simulink model "c00009M_harness"  (R2018a)
settings: Solver=FixedStepAuto  StartTime=0.0  StopTime=300  FixedStep=0.1  RelTol=1e-3
undefined symbols (not defined in the file): A1, hmax, PriorityTank, R1, R2, sigbuilder_block
(part 8 of 29)

== system c00009M_harness/M090/Tank2 ==
  CT2 : Inport
  MR2 : Inport  Port=2
  T2 : Inport  Port=3
  EB2 : Inport  Port=4
  LL1 : Inport  Port=5
  Control : Subsystem
  Logical Operator : Logic  AllPortsSameDT=off  OutDataTypeStr=boolean
  MasterTankControl : Subsystem
  Memory : Memory
  Memory1 : Memory
  TankModel : Subsystem
  LL2 : Outport
  wires:
  TankModel/1(LiquidLevel) -> Memory/1, LL2/1
  Control/1(LiquidIn) -> Logical Operator/1
  Control/2(LiquidOut) -> TankModel/2(LiquidOut)
  Memory/1 -> Control/5(LiquidLevel), MasterTankControl/2(LiquidTank2)
  MR2/1 -> Control/3(ManualReference)
  CT2/1 -> Control/2(StartMaintenance), Control/1(ControlType)
  Memory1/1 -> MasterTankControl/1(LiquidTank1)
  EB2/1 -> Control/4(EmergencyButton)
  MasterTankControl/1(AllowTheTankFilling) -> Logical Operator/2
  Logical Operator/1 -> TankModel/1(LiquidIn)
  LL1/1 -> Memory1/1

== system c00009M_harness/M091/Tank1 ==
  CT1 : Inport
  MR1 : Inport  Port=2
  T1 : Inport  Port=3
  EB1 : Inport  Port=4
  LL2 : Inport  Port=5
  Control : Subsystem
  Logical Operator : Logic  AllPortsSameDT=off  OutDataTypeStr=boolean
  MasterTankControl : Subsystem
  Memory : Memory
  Memory1 : Memory
  TankModel : Subsystem
  LL1 : Outport
  wires:
  TankModel/1(LiquidLevel) -> Memory/1, LL1/1
  Control/1(LiquidIn) -> Logical Operator/1
  Control/2(LiquidOut) -> TankModel/2(LiquidOut)
  Memory/1 -> Control/4(LiquidLevel), MasterTankControl/1(LiquidTank1)
  MR1/1 -> Control/2(ManualReference)
  CT1/1 -> Control/1(ControlType)
  Memory1/1 -> MasterTankControl/2(LiquidTank2)
  EB1/1 -> Control/3(EmergencyButton)
  MasterTankControl/1(AllowTheTankFilling) -> Logical Operator/2
  Logical Operator/1 -> TankModel/1(LiquidIn)
  LL2/1 -> Memory1/1

== system c00009M_harness/M091/Tank2 ==
  CT2 : Inport
  MR2 : Inport  Port=2
  T2 : Inport  Port=3
  EB2 : Inport  Port=4
  LL1 : Inport  Port=5
  Control : Subsystem
  Logical Operator : Logic  AllPortsSameDT=off  OutDataTypeStr=boolean
  MasterTankControl : Subsystem
  Memory : Memory
  Memory1 : Memory
  TankModel : Subsystem
  LL2 : Outport
  wires:
  TankModel/1(LiquidLevel) -> Memory/1, LL2/1
  Control/1(LiquidIn) -> Logical Operator/1
  Control/2(LiquidOut) -> TankModel/2(LiquidOut)
  Memory/1 -> Control/5(LiquidLevel), MasterTankControl/2(LiquidTank2)
  MR2/1 -> Control/3(ManualReference)
  CT2/1 -> Control/2(StartMaintenance), Control/1(ControlType)
  Memory1/1 -> MasterTankControl/1(LiquidTank1)
  EB2/1 -> Control/4(EmergencyButton)
  MasterTankControl/1(AllowTheTankFilling) -> Logical Operator/2
  Logical Operator/1 -> TankModel/1(LiquidIn)
  LL1/1 -> Memory1/1

== system c00009M_harness/M092/Tank1 ==
  CT1 : Inport
  MR1 : Inport  Port=2
  T1 : Inport  Port=3
  EB1 : Inport  Port=4
  LL2 : Inport  Port=5
  Control : Subsystem
  Logical Operator : Logic  AllPortsSameDT=off  OutDataTypeStr=boolean
  MasterTankControl : Subsystem
  Memory : Memory
  Memory1 : Memory
  TankModel : Subsystem
  LL1 : Outport
  wires:
  TankModel/1(LiquidLevel) -> Memory/1, LL1/1
  Control/1(LiquidIn) -> Logical Operator/1
  Control/2(LiquidOut) -> TankModel/2(LiquidOut)
  Memory/1 -> Control/4(LiquidLevel), MasterTankControl/1(LiquidTank1)
  MR1/1 -> Control/2(ManualReference)
  CT1/1 -> Control/1(ControlType)
  Memory1/1 -> MasterTankControl/2(LiquidTank2)
  EB1/1 -> Control/3(EmergencyButton)
  MasterTankControl/1(AllowTheTankFilling) -> Logical Operator/2
  Logical Operator/1 -> TankModel/1(LiquidIn)
  LL2/1 -> Memory1/1

== system c00009M_harness/M092/Tank2 ==
  CT2 : Inport
  MR2 : Inport  Port=2
  T2 : Inport  Port=3
  EB2 : Inport  Port=4
  LL1 : Inport  Port=5
  Control : Subsystem
  Logical Operator : Logic  AllPortsSameDT=off  OutDataTypeStr=boolean
  MasterTankControl : Subsystem
  Memory : Memory
  Memory1 : Memory
  TankModel : Subsystem
  LL2 : Outport
  wires:
  TankModel/1(LiquidLevel) -> Memory/1, LL2/1
  Control/1(LiquidIn) -> Logical Operator/1
  Control/2(LiquidOut) -> TankModel/2(LiquidOut)
  Memory/1 -> Control/5(LiquidLevel), MasterTankControl/2(LiquidTank2)
  MR2/1 -> Control/3(ManualReference)
  CT2/1 -> Control/2(StartMaintenance), Control/1(ControlType)
  Memory1/1 -> MasterTankControl/1(LiquidTank1)
  EB2/1 -> Control/4(EmergencyButton)
  MasterTankControl/1(AllowTheTankFilling) -> Logical Operator/2
  Logical Operator/1 -> TankModel/1(LiquidIn)
  LL1/1 -> Memory1/1

== system c00009M_harness/M093/Tank1 ==
  CT1 : Inport
  MR1 : Inport  Port=2
  T1 : Inport  Port=3
  EB1 : Inport  Port=4
  LL2 : Inport  Port=5
  Control : Subsystem
  Logical Operator : Logic  AllPortsSameDT=off  OutDataTypeStr=boolean
  MasterTankControl : Subsystem
  Memory : Memory
  Memory1 : Memory
  TankModel : Subsystem
  LL1 : Outport
  wires:
  TankModel/1(LiquidLevel) -> Memory/1, LL1/1
  Control/1(LiquidIn) -> Logical Operator/1
  Control/2(LiquidOut) -> TankModel/2(LiquidOut)
  Memory/1 -> Control/4(LiquidLevel), MasterTankControl/1(LiquidTank1)
  MR1/1 -> Control/2(ManualReference)
  CT1/1 -> Control/1(ControlType)
  Memory1/1 -> MasterTankControl/2(LiquidTank2)
  EB1/1 -> Control/3(EmergencyButton)
  MasterTankControl/1(AllowTheTankFilling) -> Logical Operator/2
  Logical Operator/1 -> TankModel/1(LiquidIn)
  LL2/1 -> Memory1/1

== system c00009M_harness/M093/Tank2 ==
  CT2 : Inport
  MR2 : Inport  Port=2
  T2 : Inport  Port=3
  EB2 : Inport  Port=4
  LL1 : Inport  Port=5
  Control : Subsystem
  Logical Operator : Logic  AllPortsSameDT=off  OutDataTypeStr=boolean
  MasterTankControl : Subsystem
  Memory : Memory
  Memory1 : Memory
  TankModel : Subsystem
  LL2 : Outport
  wires:
  TankModel/1(LiquidLevel) -> Memory/1, LL2/1
  Control/1(LiquidIn) -> Logical Operator/1
  Control/2(LiquidOut) -> TankModel/2(LiquidOut)
  Memory/1 -> Control/5(LiquidLevel), MasterTankControl/2(LiquidTank2)
  MR2/1 -> Control/3(ManualReference)
  CT2/1 -> Control/2(StartMaintenance), Control/1(ControlType)
  Memory1/1 -> MasterTankControl/1(LiquidTank1)
  EB2/1 -> Control/4(EmergencyButton)
  MasterTankControl/1(AllowTheTankFilling) -> Logical Operator/2
  Logical Operator/1 -> TankModel/1(LiquidIn)
  LL1/1 -> Memory1/1

== system c00009M_harness/M094/Tank1 ==
  CT1 : Inport
  MR1 : Inport  Port=2
  T1 : Inport  Port=3
  EB1 : Inport  Port=4
  LL2 : Inport  Port=5
  Control : Subsystem
  Logical Operator : Logic  AllPortsSameDT=off  OutDataTypeStr=boolean
  MasterTankControl : Subsystem
  Memory : Memory
  Memory1 : Memory
  TankModel : Subsystem
  LL1 : Outport
  wires:
  TankModel/1(LiquidLevel) -> Memory/1, LL1/1
  Control/1(LiquidIn) -> Logical Operator/1
  Control/2(LiquidOut) -> TankModel/2(LiquidOut)
  Memory/1 -> Control/4(LiquidLevel), MasterTankControl/1(LiquidTank1)
  MR1/1 -> Control/2(ManualReference)
  CT1/1 -> Control/1(ControlType)
  Memory1/1 -> MasterTankControl/2(LiquidTank2)
  EB1/1 -> Control/3(EmergencyButton)
  MasterTankControl/1(AllowTheTankFilling) -> Logical Operator/2
  Logical Operator/1 -> TankModel/1(LiquidIn)
  LL2/1 -> Memory1/1

== system c00009M_harness/M094/Tank2 ==
  CT2 : Inport
  MR2 : Inport  Port=2
  T2 : Inport  Port=3
  EB2 : Inport  Port=4
  LL1 : Inport  Port=5
  Control : Subsystem
  Logical Operator : Logic  AllPortsSameDT=off  OutDataTypeStr=boolean
  MasterTankControl : Subsystem
  Memory : Memory
  Memory1 : Memory
  TankModel : Subsystem
  LL2 : Outport
  wires:
  TankModel/1(LiquidLevel) -> Memory/1, LL2/1
  Control/1(LiquidIn) -> Logical Operator/1
  Control/2(LiquidOut) -> TankModel/2(LiquidOut)
  Memory/1 -> Control/5(LiquidLevel), MasterTankControl/2(LiquidTank2)
  MR2/1 -> Control/3(ManualReference)
  CT2/1 -> Control/2(StartMaintenance), Control/1(ControlType)
  Memory1/1 -> MasterTankControl/1(LiquidTank1)
  EB2/1 -> Control/4(EmergencyButton)
  MasterTankControl/1(AllowTheTankFilling) -> Logical Operator/2
  Logical Operator/1 -> TankModel/1(LiquidIn)
  LL1/1 -> Memory1/1

== system c00009M_harness/M095/Tank1 ==
  CT1 : Inport
  MR1 : Inport  Port=2
  T1 : Inport  Port=3
  EB1 : Inport  Port=4
  LL2 : Inport  Port=5
  Control : Subsystem
  Logical Operator : Logic  AllPortsSameDT=off  OutDataTypeStr=boolean
  MasterTankControl : Subsystem
  Memory : Memory
  Memory1 : Memory
  TankModel : Subsystem
  LL1 : Outport
  wires:
  TankModel/1(LiquidLevel) -> Memory/1, LL1/1
  Control/1(LiquidIn) -> Logical Operator/1
  Control/2(LiquidOut) -> TankModel/2(LiquidOut)
  Memory/1 -> Control/4(LiquidLevel), MasterTankControl/1(LiquidTank1)
  MR1/1 -> Control/2(ManualReference)
  CT1/1 -> Control/1(ControlType)
  Memory1/1 -> MasterTankControl/2(LiquidTank2)
  EB1/1 -> Control/3(EmergencyButton)
  MasterTankControl/1(AllowTheTankFilling) -> Logical Operator/2
  Logical Operator/1 -> TankModel/1(LiquidIn)
  LL2/1 -> Memory1/1

== system c00009M_harness/M095/Tank2 ==
  CT2 : Inport
  MR2 : Inport  Port=2
  T2 : Inport  Port=3
  EB2 : Inport  Port=4
  LL1 : Inport  Port=5
  Control : Subsystem
  Logical Operator : Logic  AllPortsSameDT=off  OutDataTypeStr=boolean
  MasterTankControl : Subsystem
  Memory : Memory
  Memory1 : Memory
  TankModel : Subsystem
  LL2 : Outport
  wires:
  TankModel/1(LiquidLevel) -> Memory/1, LL2/1
  Control/1(LiquidIn) -> Logical Operator/1
  Control/2(LiquidOut) -> TankModel/2(LiquidOut)
  Memory/1 -> Control/5(LiquidLevel), MasterTankControl/2(LiquidTank2)
  MR2/1 -> Control/3(ManualReference)
  CT2/1 -> Control/2(StartMaintenance), Control/1(ControlType)
  Memory1/1 -> MasterTankControl/1(LiquidTank1)
  EB2/1 -> Control/4(EmergencyButton)
  MasterTankControl/1(AllowTheTankFilling) -> Logical Operator/2
  Logical Operator/1 -> TankModel/1(LiquidIn)
  LL1/1 -> Memory1/1

== system c00009M_harness/M096/Tank1 ==
  CT1 : Inport
  MR1 : Inport  Port=2
  T1 : Inport  Port=3
  EB1 : Inport  Port=4
  LL2 : Inport  Port=5
  Control : Subsystem
  Logical Operator : Logic  AllPortsSameDT=off  OutDataTypeStr=boolean
  MasterTankControl : Subsystem
  Memory : Memory
  Memory1 : Memory
  TankModel : Subsystem
  LL1 : Outport
  wires:
  TankModel/1(LiquidLevel) -> Memory/1, LL1/1
  Control/1(LiquidIn) -> Logical Operator/1
  Control/2(LiquidOut) -> TankModel/2(LiquidOut)
  Memory/1 -> Control/4(LiquidLevel), MasterTankControl/1(LiquidTank1)
  MR1/1 -> Control/2(ManualReference)
  CT1/1 -> Control/1(ControlType)
  Memory1/1 -> MasterTankControl/2(LiquidTank2)
  EB1/1 -> Control/3(EmergencyButton)
  MasterTankControl/1(AllowTheTankFilling) -> Logical Operator/2
  Logical Operator/1 -> TankModel/1(LiquidIn)
  LL2/1 -> Memory1/1

== system c00009M_harness/M096/Tank2 ==
  CT2 : Inport
  MR2 : Inport  Port=2
  T2 : Inport  Port=3
  EB2 : Inport  Port=4
  LL1 : Inport  Port=5
  Control : Subsystem
  Logical Operator : Logic  AllPortsSameDT=off  OutDataTypeStr=boolean
  MasterTankControl : Subsystem
  Memory : Memory
  Memory1 : Memory
  TankModel : Subsystem
  LL2 : Outport
  wires:
  TankModel/1(LiquidLevel) -> Memory/1, LL2/1
  Control/1(LiquidIn) -> Logical Operator/1
  Control/2(LiquidOut) -> TankModel/2(LiquidOut)
  Memory/1 -> Control/5(LiquidLevel), MasterTankControl/2(LiquidTank2)
  MR2/1 -> Control/3(ManualReference)
  CT2/1 -> Control/2(StartMaintenance), Control/1(ControlType)
  Memory1/1 -> MasterTankControl/1(LiquidTank1)
  EB2/1 -> Control/4(EmergencyButton)
  MasterTankControl/1(AllowTheTankFilling) -> Logical Operator/2
  Logical Operator/1 -> TankModel/1(LiquidIn)
  LL1/1 -> Memory1/1

== system c00009M_harness/M097/Tank1 ==
  CT1 : Inport
  MR1 : Inport  Port=2
  T1 : Inport  Port=3
  EB1 : Inport  Port=4
  LL2 : Inport  Port=5
  Control : Subsystem
  Logical Operator : Logic  AllPortsSameDT=off  OutDataTypeStr=boolean
  MasterTankControl : Subsystem
  Memory : Memory
  Memory1 : Memory
  TankModel : Subsystem
  LL1 : Outport
  wires:
  TankModel/1(LiquidLevel) -> Memory/1, LL1/1
  Control/1(LiquidIn) -> Logical Operator/1
  Control/2(LiquidOut) -> TankModel/2(LiquidOut)
  Memory/1 -> Control/4(LiquidLevel), MasterTankControl/1(LiquidTank1)
  MR1/1 -> Control/2(ManualReference)
  CT1/1 -> Control/1(ControlType)
  Memory1/1 -> MasterTankControl/2(LiquidTank2)
  EB1/1 -> Control/3(EmergencyButton)
  MasterTankControl/1(AllowTheTankFilling) -> Logical Operator/2
  Logical Operator/1 -> TankModel/1(LiquidIn)
  LL2/1 -> Memory1/1

== system c00009M_harness/M097/Tank2 ==
  CT2 : Inport
  MR2 : Inport  Port=2
  T2 : Inport  Port=3
  EB2 : Inport  Port=4
  LL1 : Inport  Port=5
  Control : Subsystem
  Logical Operator : Logic  AllPortsSameDT=off  OutDataTypeStr=boolean
  MasterTankControl : Subsystem
  Memory : Memory
  Memory1 : Memory
  TankModel : Subsystem
  LL2 : Outport
  wires:
  TankModel/1(LiquidLevel) -> Memory/1, LL2/1
  Control/1(LiquidIn) -> Logical Operator/1
  Control/2(LiquidOut) -> TankModel/2(LiquidOut)
  Memory/1 -> Control/5(LiquidLevel), MasterTankControl/2(LiquidTank2)
  MR2/1 -> Control/3(ManualReference)
  CT2/1 -> Control/2(StartMaintenance), Control/1(ControlType)
  Memory1/1 -> MasterTankControl/1(LiquidTank1)
  EB2/1 -> Control/4(EmergencyButton)
  MasterTankControl/1(AllowTheTankFilling) -> Logical Operator/2
  Logical Operator/1 -> TankModel/1(LiquidIn)
  LL1/1 -> Memory1/1

== system c00009M_harness/M098/Tank1 ==
  CT1 : Inport
  MR1 : Inport  Port=2
  T1 : Inport  Port=3
  EB1 : Inport  Port=4
  LL2 : Inport  Port=5
  Control : Subsystem
  Logical Operator : Logic  AllPortsSameDT=off  OutDataTypeStr=boolean
  MasterTankControl : Subsystem
  Memory : Memory
  Memory1 : Memory
  TankModel : Subsystem
  LL1 : Outport
  wires:
  TankModel/1(LiquidLevel) -> Memory/1, LL1/1
  Control/1(LiquidIn) -> Logical Operator/1
  Control/2(LiquidOut) -> TankModel/2(LiquidOut)
  Memory/1 -> Control/4(LiquidLevel), MasterTankControl/1(LiquidTank1)
  MR1/1 -> Control/2(ManualReference)
  CT1/1 -> Control/1(ControlType)
  Memory1/1 -> MasterTankControl/2(LiquidTank2)
  EB1/1 -> Control/3(EmergencyButton)
  MasterTankControl/1(AllowTheTankFilling) -> Logical Operator/2
  Logical Operator/1 -> TankModel/1(LiquidIn)
  LL2/1 -> Memory1/1

== system c00009M_harness/M098/Tank2 ==
  CT2 : Inport
  MR2 : Inport  Port=2
  T2 : Inport  Port=3
  EB2 : Inport  Port=4
  LL1 : Inport  Port=5
  Control : Subsystem
  Logical Operator : Logic  AllPortsSameDT=off  OutDataTypeStr=boolean
  MasterTankControl : Subsystem
  Memory : Memory
  Memory1 : Memory
  TankModel : Subsystem
  LL2 : Outport
  wires:
  TankModel/1(LiquidLevel) -> Memory/1, LL2/1
  Control/1(LiquidIn) -> Logical Operator/1
  Control/2(LiquidOut) -> TankModel/2(LiquidOut)
  Memory/1 -> Control/5(LiquidLevel), MasterTankControl/2(LiquidTank2)
  MR2/1 -> Control/3(ManualReference)
  CT2/1 -> Control/2(StartMaintenance), Control/1(ControlType)
  Memory1/1 -> MasterTankControl/1(LiquidTank1)
  EB2/1 -> Control/4(EmergencyButton)
  MasterTankControl/1(AllowTheTankFilling) -> Logical Operator/2
  Logical Operator/1 -> TankModel/1(LiquidIn)
  LL1/1 -> Memory1/1

== system c00009M_harness/M099/Tank1 ==
  CT1 : Inport
  MR1 : Inport  Port=2
  T1 : Inport  Port=3
  EB1 : Inport  Port=4
  LL2 : Inport  Port=5
  Control : Subsystem
  Logical Operator : Logic  AllPortsSameDT=off  OutDataTypeStr=boolean
  MasterTankControl : Subsystem
  Memory : Memory
  Memory1 : Memory
  TankModel : Subsystem
  LL1 : Outport
  wires:
  TankModel/1(LiquidLevel) -> Memory/1, LL1/1
  Control/1(LiquidIn) -> Logical Operator/1
  Control/2(LiquidOut) -> TankModel/2(LiquidOut)
  Memory/1 -> Control/4(LiquidLevel), MasterTankControl/1(LiquidTank1)
  MR1/1 -> Control/2(ManualReference)
  CT1/1 -> Control/1(ControlType)
  Memory1/1 -> MasterTankControl/2(LiquidTank2)
  EB1/1 -> Control/3(EmergencyButton)
  MasterTankControl/1(AllowTheTankFilling) -> Logical Operator/2
  Logical Operator/1 -> TankModel/1(LiquidIn)
  LL2/1 -> Memory1/1

== system c00009M_harness/M099/Tank2 ==
  CT2 : Inport
  MR2 : Inport  Port=2
  T2 : Inport  Port=3
  EB2 : Inport  Port=4
  LL1 : Inport  Port=5
  Control : Subsystem
  Logical Operator : Logic  AllPortsSameDT=off  OutDataTypeStr=boolean
  MasterTankControl : Subsystem
  Memory : Memory
  Memory1 : Memory
  TankModel : Subsystem
  LL2 : Outport
  wires:
  TankModel/1(LiquidLevel) -> Memory/1, LL2/1
  Control/1(LiquidIn) -> Logical Operator/1
  Control/2(LiquidOut) -> TankModel/2(LiquidOut)
  Memory/1 -> Control/5(LiquidLevel), MasterTankControl/2(LiquidTank2)
  MR2/1 -> Control/3(ManualReference)
  CT2/1 -> Control/2(StartMaintenance), Control/1(ControlType)
  Memory1/1 -> MasterTankControl/1(LiquidTank1)
  EB2/1 -> Control/4(EmergencyButton)
  MasterTankControl/1(AllowTheTankFilling) -> Logical Operator/2
  Logical Operator/1 -> TankModel/1(LiquidIn)
  LL1/1 -> Memory1/1

== system c00009M_harness/M100/Tank1 ==
  CT1 : Inport
  MR1 : Inport  Port=2
  T1 : Inport  Port=3
  EB1 : Inport  Port=4
  LL2 : Inport  Port=5
  Control : Subsystem
  Logical Operator : Logic  AllPortsSameDT=off  OutDataTypeStr=boolean
  MasterTankControl : Subsystem
  Memory : Memory
  Memory1 : Memory
  TankModel : Subsystem
  LL1 : Outport
  wires:
  TankModel/1(LiquidLevel) -> Memory/1, LL1/1
  Control/1(LiquidIn) -> Logical Operator/1
  Control/2(LiquidOut) -> TankModel/2(LiquidOut)
  Memory/1 -> Control/4(LiquidLevel), MasterTankControl/1(LiquidTank1)
  MR1/1 -> Control/2(ManualReference)
  CT1/1 -> Control/1(ControlType)
  Memory1/1 -> MasterTankControl/2(LiquidTank2)
  EB1/1 -> Control/3(EmergencyButton)
  MasterTankControl/1(AllowTheTankFilling) -> Logical Operator/2
  Logical Operator/1 -> TankModel/1(LiquidIn)
  LL2/1 -> Memory1/1

== system c00009M_harness/M100/Tank2 ==
  CT2 : Inport
  MR2 : Inport  Port=2
  T2 : Inport  Port=3
  EB2 : Inport  Port=4
  LL1 : Inport  Port=5
  Control : Subsystem
  Logical Operator : Logic  AllPortsSameDT=off  OutDataTypeStr=boolean
  MasterTankControl : Subsystem
  Memory : Memory
  Memory1 : Memory
  TankModel : Subsystem
  LL2 : Outport
  wires:
  TankModel/1(LiquidLevel) -> Memory/1, LL2/1
  Control/1(LiquidIn) -> Logical Operator/1
  Control/2(LiquidOut) -> TankModel/2(LiquidOut)
  Memory/1 -> Control/5(LiquidLevel), MasterTankControl/2(LiquidTank2)
  MR2/1 -> Control/3(ManualReference)
  CT2/1 -> Control/2(StartMaintenance), Control/1(ControlType)
  Memory1/1 -> MasterTankControl/1(LiquidTank1)
  EB2/1 -> Control/4(EmergencyButton)
  MasterTankControl/1(AllowTheTankFilling) -> Logical Operator/2
  Logical Operator/1 -> TankModel/1(LiquidIn)
  LL1/1 -> Memory1/1

== system c00009M_harness/M101/Tank1 ==
  CT1 : Inport
  MR1 : Inport  Port=2
  T1 : Inport  Port=3
  EB1 : Inport  Port=4
  LL2 : Inport  Port=5
  Control : Subsystem
  Logical Operator : Logic  AllPortsSameDT=off  OutDataTypeStr=boolean
  MasterTankControl : Subsystem
  Memory : Memory
  Memory1 : Memory
  TankModel : Subsystem
  LL1 : Outport
  wires:
  TankModel/1(LiquidLevel) -> Memory/1, LL1/1
  Control/1(LiquidIn) -> Logical Operator/1
  Control/2(LiquidOut) -> TankModel/2(LiquidOut)
  Memory/1 -> Control/4(LiquidLevel), MasterTankControl/1(LiquidTank1)
  MR1/1 -> Control/2(ManualReference)
  CT1/1 -> Control/1(ControlType)
  Memory1/1 -> MasterTankControl/2(LiquidTank2)
  EB1/1 -> Control/3(EmergencyButton)
  MasterTankControl/1(AllowTheTankFilling) -> Logical Operator/2
  Logical Operator/1 -> TankModel/1(LiquidIn)
  LL2/1 -> Memory1/1

== system c00009M_harness/M101/Tank2 ==
  CT2 : Inport
  MR2 : Inport  Port=2
  T2 : Inport  Port=3
  EB2 : Inport  Port=4
  LL1 : Inport  Port=5
  Control : Subsystem
  Logical Operator : Logic  AllPortsSameDT=off  OutDataTypeStr=boolean
  MasterTankControl : Subsystem
  Memory : Memory
  Memory1 : Memory
  TankModel : Subsystem
  LL2 : Outport
  wires:
  TankModel/1(LiquidLevel) -> Memory/1, LL2/1
  Control/1(LiquidIn) -> Logical Operator/1
  Control/2(LiquidOut) -> TankModel/2(LiquidOut)
  Memory/1 -> Control/5(LiquidLevel), MasterTankControl/2(LiquidTank2)
  MR2/1 -> Control/3(ManualReference)
  CT2/1 -> Control/2(StartMaintenance), Control/1(ControlType)
  Memory1/1 -> MasterTankControl/1(LiquidTank1)
  EB2/1 -> Control/4(EmergencyButton)
  MasterTankControl/1(AllowTheTankFilling) -> Logical Operator/2
  Logical Operator/1 -> TankModel/1(LiquidIn)
  LL1/1 -> Memory1/1

== system c00009M_harness/M102/Tank1 ==
  CT1 : Inport
  MR1 : Inport  Port=2
  T1 : Inport  Port=3
  EB1 : Inport  Port=4
  LL2 : Inport  Port=5
  Control : Subsystem
  Logical Operator : Logic  AllPortsSameDT=off  OutDataTypeStr=boolean
  MasterTankControl : Subsystem
  Memory : Memory
  Memory1 : Memory
  TankModel : Subsystem
  LL1 : Outport
  wires:
  TankModel/1(LiquidLevel) -> Memory/1, LL1/1
  Control/1(LiquidIn) -> Logical Operator/1
  Control/2(LiquidOut) -> TankModel/2(LiquidOut)
  Memory/1 -> Control/4(LiquidLevel), MasterTankControl/1(LiquidTank1)
  MR1/1 -> Control/2(ManualReference)
  CT1/1 -> Control/1(ControlType)
  Memory1/1 -> MasterTankControl/2(LiquidTank2)
  EB1/1 -> Control/3(EmergencyButton)
  MasterTankControl/1(AllowTheTankFilling) -> Logical Operator/2
  Logical Operator/1 -> TankModel/1(LiquidIn)
  LL2/1 -> Memory1/1

== system c00009M_harness/M102/Tank2 ==
  CT2 : Inport
  MR2 : Inport  Port=2
  T2 : Inport  Port=3
  EB2 : Inport  Port=4
  LL1 : Inport  Port=5
  Control : Subsystem
  Logical Operator : Logic  AllPortsSameDT=off  OutDataTypeStr=boolean
  MasterTankControl : Subsystem
  Memory : Memory
  Memory1 : Memory
  TankModel : Subsystem
  LL2 : Outport
  wires:
  TankModel/1(LiquidLevel) -> Memory/1, LL2/1
  Control/1(LiquidIn) -> Logical Operator/1
  Control/2(LiquidOut) -> TankModel/2(LiquidOut)
  Memory/1 -> Control/5(LiquidLevel), MasterTankControl/2(LiquidTank2)
  MR2/1 -> Control/3(ManualReference)
  CT2/1 -> Control/2(StartMaintenance), Control/1(ControlType)
  Memory1/1 -> MasterTankControl/1(LiquidTank1)
  EB2/1 -> Control/4(EmergencyButton)
  MasterTankControl/1(AllowTheTankFilling) -> Logical Operator/2
  Logical Operator/1 -> TankModel/1(LiquidIn)
  LL1/1 -> Memory1/1

== system c00009M_harness/M103/Tank1 ==
  CT1 : Inport
  MR1 : Inport  Port=2
  T1 : Inport  Port=3
  EB1 : Inport  Port=4
  LL2 : Inport  Port=5
  Control : Subsystem
  Logical Operator : Logic  AllPortsSameDT=off  OutDataTypeStr=boolean
  MasterTankControl : Subsystem
  Memory : Memory
  Memory1 : Memory
  TankModel : Subsystem
  LL1 : Outport
  wires:
  TankModel/1(LiquidLevel) -> Memory/1, LL1/1
  Control/1(LiquidIn) -> Logical Operator/1
  Control/2(LiquidOut) -> TankModel/2(LiquidOut)
  Memory/1 -> Control/4(LiquidLevel), MasterTankControl/1(LiquidTank1)
  MR1/1 -> Control/2(ManualReference)
  CT1/1 -> Control/1(ControlType)
  Memory1/1 -> MasterTankControl/2(LiquidTank2)
  EB1/1 -> Control/3(EmergencyButton)
  MasterTankControl/1(AllowTheTankFilling) -> Logical Operator/2
  Logical Operator/1 -> TankModel/1(LiquidIn)
  LL2/1 -> Memory1/1

== system c00009M_harness/M103/Tank2 ==
  CT2 : Inport
  MR2 : Inport  Port=2
  T2 : Inport  Port=3
  EB2 : Inport  Port=4
  LL1 : Inport  Port=5
  Control : Subsystem
  Logical Operator : Logic  AllPortsSameDT=off  OutDataTypeStr=boolean
  MasterTankControl : Subsystem
  Memory : Memory
  Memory1 : Memory
  TankModel : Subsystem
  LL2 : Outport
  wires:
  TankModel/1(LiquidLevel) -> Memory/1, LL2/1
  Control/1(LiquidIn) -> Logical Operator/1
  Control/2(LiquidOut) -> TankModel/2(LiquidOut)
  Memory/1 -> Control/5(LiquidLevel), MasterTankControl/2(LiquidTank2)
  MR2/1 -> Control/3(ManualReference)
  CT2/1 -> Control/2(StartMaintenance), Control/1(ControlType)
  Memory1/1 -> MasterTankControl/1(LiquidTank1)
  EB2/1 -> Control/4(EmergencyButton)
  MasterTankControl/1(AllowTheTankFilling) -> Logical Operator/2
  Logical Operator/1 -> TankModel/1(LiquidIn)
  LL1/1 -> Memory1/1

== system c00009M_harness/M104/Tank1 ==
  CT1 : Inport
  MR1 : Inport  Port=2
  T1 : Inport  Port=3
  EB1 : Inport  Port=4
  LL2 : Inport  Port=5
  Control : Subsystem
  Logical Operator : Logic  AllPortsSameDT=off  OutDataTypeStr=boolean
  MasterTankControl : Subsystem
  Memory : Memory
  Memory1 : Memory
  TankModel : Subsystem
  LL1 : Outport
  wires:
  TankModel/1(LiquidLevel) -> Memory/1, LL1/1
  Control/1(LiquidIn) -> Logical Operator/1
  Control/2(LiquidOut) -> TankModel/2(LiquidOut)
  Memory/1 -> Control/4(LiquidLevel), MasterTankControl/1(LiquidTank1)
  MR1/1 -> Control/2(ManualReference)
  CT1/1 -> Control/1(ControlType)
  Memory1/1 -> MasterTankControl/2(LiquidTank2)
  EB1/1 -> Control/3(EmergencyButton)
  MasterTankControl/1(AllowTheTankFilling) -> Logical Operator/2
  Logical Operator/1 -> TankModel/1(LiquidIn)
  LL2/1 -> Memory1/1

== system c00009M_harness/M104/Tank2 ==
  CT2 : Inport
  MR2 : Inport  Port=2
  T2 : Inport  Port=3
  EB2 : Inport  Port=4
  LL1 : Inport  Port=5
  Control : Subsystem
  Logical Operator : Logic  AllPortsSameDT=off  OutDataTypeStr=boolean
  MasterTankControl : Subsystem
  Memory : Memory
  Memory1 : Memory
  TankModel : Subsystem
  LL2 : Outport
  wires:
  TankModel/1(LiquidLevel) -> Memory/1, LL2/1
  Control/1(LiquidIn) -> Logical Operator/1
  Control/2(LiquidOut) -> TankModel/2(LiquidOut)
  Memory/1 -> Control/5(LiquidLevel), MasterTankControl/2(LiquidTank2)
  MR2/1 -> Control/3(ManualReference)
  CT2/1 -> Control/2(StartMaintenance), Control/1(ControlType)
  Memory1/1 -> MasterTankControl/1(LiquidTank1)
  EB2/1 -> Control/4(EmergencyButton)
  MasterTankControl/1(AllowTheTankFilling) -> Logical Operator/2
  Logical Operator/1 -> TankModel/1(LiquidIn)
  LL1/1 -> Memory1/1

== system c00009M_harness/M105/Tank1 ==
  CT1 : Inport
  MR1 : Inport  Port=2
  T1 : Inport  Port=3
  EB1 : Inport  Port=4
  LL2 : Inport  Port=5
  Control : Subsystem
  Logical Operator : Logic  AllPortsSameDT=off  OutDataTypeStr=boolean
  MasterTankControl : Subsystem
  Memory : Memory
  Memory1 : Memory
  TankModel : Subsystem
  LL1 : Outport
  wires:
  TankModel/1(LiquidLevel) -> Memory/1, LL1/1
  Control/1(LiquidIn) -> Logical Operator/1
  Control/2(LiquidOut) -> TankModel/2(LiquidOut)
  Memory/1 -> Control/4(LiquidLevel), MasterTankControl/1(LiquidTank1)
  MR1/1 -> Control/2(ManualReference)
  CT1/1 -> Control/1(ControlType)
  Memory1/1 -> MasterTankControl/2(LiquidTank2)
  EB1/1 -> Control/3(EmergencyButton)
  MasterTankControl/1(AllowTheTankFilling) -> Logical Operator/2
  Logical Operator/1 -> TankModel/1(LiquidIn)
  LL2/1 -> Memory1/1

== system c00009M_harness/M105/Tank2 ==
  CT2 : Inport
  MR2 : Inport  Port=2
  T2 : Inport  Port=3
  EB2 : Inport  Port=4
  LL1 : Inport  Port=5
  Control : Subsystem
  Logical Operator : Logic  AllPortsSameDT=off  OutDataTypeStr=boolean
  MasterTankControl : Subsystem
  Memory : Memory
  Memory1 : Memory
  TankModel : Subsystem
  LL2 : Outport
  wires:
  TankModel/1(LiquidLevel) -> Memory/1, LL2/1
  Control/1(LiquidIn) -> Logical Operator/1
  Control/2(LiquidOut) -> TankModel/2(LiquidOut)
  Memory/1 -> Control/5(LiquidLevel), MasterTankControl/2(LiquidTank2)
  MR2/1 -> Control/3(ManualReference)
  CT2/1 -> Control/2(StartMaintenance), Control/1(ControlType)
  Memory1/1 -> MasterTankControl/1(LiquidTank1)
  EB2/1 -> Control/4(EmergencyButton)
  MasterTankControl/1(AllowTheTankFilling) -> Logical Operator/2
  Logical Operator/1 -> TankModel/1(LiquidIn)
  LL1/1 -> Memory1/1

== system c00009M_harness/M106/Tank1 ==
  CT1 : Inport
  MR1 : Inport  Port=2
  T1 : Inport  Port=3
  EB1 : Inport  Port=4
  LL2 : Inport  Port=5
  Control : Subsystem
  Logical Operator : Logic  AllPortsSameDT=off  OutDataTypeStr=boolean
  MasterTankControl : Subsystem
  Memory : Memory
  Memory1 : Memory
  TankModel : Subsystem
  LL1 : Outport
  wires:
  TankModel/1(LiquidLevel) -> Memory/1, LL1/1
  Control/1(LiquidIn) -> Logical Operator/1
  Control/2(LiquidOut) -> TankModel/2(LiquidOut)
  Memory/1 -> Control/4(LiquidLevel), MasterTankControl/1(LiquidTank1)
  MR1/1 -> Control/2(ManualReference)
  CT1/1 -> Control/1(ControlType)
  Memory1/1 -> MasterTankControl/2(LiquidTank2)
  EB1/1 -> Control/3(EmergencyButton)
  MasterTankControl/1(AllowTheTankFilling) -> Logical Operator/2
  Logical Operator/1 -> TankModel/1(LiquidIn)
  LL2/1 -> Memory1/1

== system c00009M_harness/M106/Tank2 ==
  CT2 : Inport
  MR2 : Inport  Port=2
  T2 : Inport  Port=3
  EB2 : Inport  Port=4
  LL1 : Inport  Port=5
  Control : Subsystem
  Logical Operator : Logic  AllPortsSameDT=off  OutDataTypeStr=boolean
  MasterTankControl : Subsystem
  Memory : Memory
  Memory1 : Memory
  TankModel : Subsystem
  LL2 : Outport
  wires:
  TankModel/1(LiquidLevel) -> Memory/1, LL2/1
  Control/1(LiquidIn) -> Logical Operator/1
  Control/2(LiquidOut) -> TankModel/2(LiquidOut)
  Memory/1 -> Control/5(LiquidLevel), MasterTankControl/2(LiquidTank2)
  MR2/1 -> Control/3(ManualReference)
  CT2/1 -> Control/2(StartMaintenance), Control/1(ControlType)
  Memory1/1 -> MasterTankControl/1(LiquidTank1)
  EB2/1 -> Control/4(EmergencyButton)
  MasterTankControl/1(AllowTheTankFilling) -> Logical Operator/2
  Logical Operator/1 -> TankModel/1(LiquidIn)
  LL1/1 -> Memory1/1

== system c00009M_harness/M107/Tank1 ==
  CT1 : Inport
  MR1 : Inport  Port=2
  T1 : Inport  Port=3
  EB1 : Inport  Port=4
  LL2 : Inport  Port=5
  Control : Subsystem
  Logical Operator : Logic  AllPortsSameDT=off  OutDataTypeStr=boolean
  MasterTankControl : Subsystem
  Memory : Memory
  Memory1 : Memory
  TankModel : Subsystem
  LL1 : Outport
  wires:
  TankModel/1(LiquidLevel) -> Memory/1, LL1/1
  Control/1(LiquidIn) -> Logical Operator/1
  Control/2(LiquidOut) -> TankModel/2(LiquidOut)
  Memory/1 -> Control/4(LiquidLevel), MasterTankControl/1(LiquidTank1)
  MR1/1 -> Control/2(ManualReference)
  CT1/1 -> Control/1(ControlType)
  Memory1/1 -> MasterTankControl/2(LiquidTank2)
  EB1/1 -> Control/3(EmergencyButton)
  MasterTankControl/1(AllowTheTankFilling) -> Logical Operator/2
  Logical Operator/1 -> TankModel/1(LiquidIn)
  LL2/1 -> Memory1/1

== system c00009M_harness/M107/Tank2 ==
  CT2 : Inport
  MR2 : Inport  Port=2
  T2 : Inport  Port=3
  EB2 : Inport  Port=4
  LL1 : Inport  Port=5
  Control : Subsystem
  Logical Operator : Logic  AllPortsSameDT=off  OutDataTypeStr=boolean
  MasterTankControl : Subsystem
  Memory : Memory
  Memory1 : Memory
  TankModel : Subsystem
  LL2 : Outport
  wires:
  TankModel/1(LiquidLevel) -> Memory/1, LL2/1
  Control/1(LiquidIn) -> Logical Operator/1
  Control/2(LiquidOut) -> TankModel/2(LiquidOut)
  Memory/1 -> Control/5(LiquidLevel), MasterTankControl/2(LiquidTank2)
  MR2/1 -> Control/3(ManualReference)
  CT2/1 -> Control/2(StartMaintenance), Control/1(ControlType)
  Memory1/1 -> MasterTankControl/1(LiquidTank1)
  EB2/1 -> Control/4(EmergencyButton)
  MasterTankControl/1(AllowTheTankFilling) -> Logical Operator/2
  Logical Operator/1 -> TankModel/1(LiquidIn)
  LL1/1 -> Memory1/1

== system c00009M_harness/M108/Tank1 ==
  CT1 : Inport
  MR1 : Inport  Port=2
  T1 : Inport  Port=3
  EB1 : Inport  Port=4
  LL2 : Inport  Port=5
  Control : Subsystem
  Logical Operator : Logic  AllPortsSameDT=off  OutDataTypeStr=boolean
  MasterTankControl : Subsystem
  Memory : Memory
  Memory1 : Memory
  TankModel : Subsystem
  LL1 : Outport
  wires:
  TankModel/1(LiquidLevel) -> Memory/1, LL1/1
  Control/1(LiquidIn) -> Logical Operator/1
  Control/2(LiquidOut) -> TankModel/2(LiquidOut)
  Memory/1 -> Control/4(LiquidLevel), MasterTankControl/1(LiquidTank1)
  MR1/1 -> Control/2(ManualReference)
  CT1/1 -> Control/1(ControlType)
  Memory1/1 -> MasterTankControl/2(LiquidTank2)
  EB1/1 -> Control/3(EmergencyButton)
  MasterTankControl/1(AllowTheTankFilling) -> Logical Operator/2
  Logical Operator/1 -> TankModel/1(LiquidIn)
  LL2/1 -> Memory1/1

== system c00009M_harness/M108/Tank2 ==
  CT2 : Inport
  MR2 : Inport  Port=2
  T2 : Inport  Port=3
  EB2 : Inport  Port=4
  LL1 : Inport  Port=5
  Control : Subsystem
  Logical Operator : Logic  AllPortsSameDT=off  OutDataTypeStr=boolean
  MasterTankControl : Subsystem
  Memory : Memory
  Memory1 : Memory
  TankModel : Subsystem
  LL2 : Outport
  wires:
  TankModel/1(LiquidLevel) -> Memory/1, LL2/1
  Control/1(LiquidIn) -> Logical Operator/1
  Control/2(LiquidOut) -> TankModel/2(LiquidOut)
  Memory/1 -> Control/5(LiquidLevel), MasterTankControl/2(LiquidTank2)
  MR2/1 -> Control/3(ManualReference)
  CT2/1 -> Control/2(StartMaintenance), Control/1(ControlType)
  Memory1/1 -> MasterTankControl/1(LiquidTank1)
  EB2/1 -> Control/4(EmergencyButton)
  MasterTankControl/1(AllowTheTankFilling) -> Logical Operator/2
  Logical Operator/1 -> TankModel/1(LiquidIn)
  LL1/1 -> Memory1/1

== system c00009M_harness/M109/Tank1 ==
  CT1 : Inport
  MR1 : Inport  Port=2
  T1 : Inport  Port=3
  EB1 : Inport  Port=4
  LL2 : Inport  Port=5
  Control : Subsystem
  Logical Operator : Logic  AllPortsSameDT=off  OutDataTypeStr=boolean
  MasterTankControl : Subsystem
  Memory : Memory
  Memory1 : Memory
  TankModel : Subsystem
  LL1 : Outport
  wires:
  TankModel/1(LiquidLevel) -> Memory/1, LL1/1
  Control/1(LiquidIn) -> Logical Operator/1
  Control/2(LiquidOut) -> TankModel/2(LiquidOut)
  Memory/1 -> Control/4(LiquidLevel), MasterTankControl/1(LiquidTank1)
  MR1/1 -> Control/2(ManualReference)
  CT1/1 -> Control/1(ControlType)
  Memory1/1 -> MasterTankControl/2(LiquidTank2)
  EB1/1 -> Control/3(EmergencyButton)
  MasterTankControl/1(AllowTheTankFilling) -> Logical Operator/2
  Logical Operator/1 -> TankModel/1(LiquidIn)
  LL2/1 -> Memory1/1

== system c00009M_harness/M109/Tank2 ==
  CT2 : Inport
  MR2 : Inport  Port=2
  T2 : Inport  Port=3
  EB2 : Inport  Port=4
  LL1 : Inport  Port=5
  Control : Subsystem
  Logical Operator : Logic  AllPortsSameDT=off  OutDataTypeStr=boolean
  MasterTankControl : Subsystem
  Memory : Memory
  Memory1 : Memory
  TankModel : Subsystem
  LL2 : Outport
  wires:
  TankModel/1(LiquidLevel) -> Memory/1, LL2/1
  Control/1(LiquidIn) -> Logical Operator/1
  Control/2(LiquidOut) -> TankModel/2(LiquidOut)
  Memory/1 -> Control/5(LiquidLevel), MasterTankControl/2(LiquidTank2)
  MR2/1 -> Control/3(ManualReference)
  CT2/1 -> Control/2(StartMaintenance), Control/1(ControlType)
  Memory1/1 -> MasterTankControl/1(LiquidTank1)
  EB2/1 -> Control/4(EmergencyButton)
  MasterTankControl/1(AllowTheTankFilling) -> Logical Operator/2
  Logical Operator/1 -> TankModel/1(LiquidIn)
  LL1/1 -> Memory1/1

== system c00009M_harness/M110/Tank1 ==
  CT1 : Inport
  MR1 : Inport  Port=2
  T1 : Inport  Port=3
  EB1 : Inport  Port=4
  LL2 : Inport  Port=5
  Control : Subsystem
  Logical Operator : Logic  AllPortsSameDT=off  OutDataTypeStr=boolean
  MasterTankControl : Subsystem
  Memory : Memory
  Memory1 : Memory
  TankModel : Subsystem
  LL1 : Outport
  wires:
  TankModel/1(LiquidLevel) -> Memory/1, LL1/1
  Control/1(LiquidIn) -> Logical Operator/1
  Control/2(LiquidOut) -> TankModel/2(LiquidOut)
  Memory/1 -> Control/4(LiquidLevel), MasterTankControl/1(LiquidTank1)
  MR1/1 -> Control/2(ManualReference)
  CT1/1 -> Control/1(ControlType)
  Memory1/1 -> MasterTankControl/2(LiquidTank2)
  EB1/1 -> Control/3(EmergencyButton)
  MasterTankControl/1(AllowTheTankFilling) -> Logical Operator/2
  Logical Operator/1 -> TankModel/1(LiquidIn)
  LL2/1 -> Memory1/1

== system c00009M_harness/M110/Tank2 ==
  CT2 : Inport
  MR2 : Inport  Port=2
  T2 : Inport  Port=3
  EB2 : Inport  Port=4
  LL1 : Inport  Port=5
  Control : Subsystem
  Logical Operator : Logic  AllPortsSameDT=off  OutDataTypeStr=boolean
  MasterTankControl : Subsystem
  Memory : Memory
  Memory1 : Memory
  TankModel : Subsystem
  LL2 : Outport
  wires:
  TankModel/1(LiquidLevel) -> Memory/1, LL2/1
  Control/1(LiquidIn) -> Logical Operator/1
  Control/2(LiquidOut) -> TankModel/2(LiquidOut)
  Memory/1 -> Control/5(LiquidLevel), MasterTankControl/2(LiquidTank2)
  MR2/1 -> Control/3(ManualReference)
  CT2/1 -> Control/2(StartMaintenance), Control/1(ControlType)
  Memory1/1 -> MasterTankControl/1(LiquidTank1)
  EB2/1 -> Control/4(EmergencyButton)
  MasterTankControl/1(AllowTheTankFilling) -> Logical Operator/2
  Logical Operator/1 -> TankModel/1(LiquidIn)
  LL1/1 -> Memory1/1

== system c00009M_harness/M111/Tank1 ==
  CT1 : Inport
  MR1 : Inport  Port=2
  T1 : Inport  Port=3
  EB1 : Inport  Port=4
  LL2 : Inport  Port=5
  Control : Subsystem
  Logical Operator : Logic  AllPortsSameDT=off  OutDataTypeStr=boolean
  MasterTankControl : Subsystem
  Memory : Memory
  Memory1 : Memory
  TankModel : Subsystem
  LL1 : Outport
  wires:
  TankModel/1(LiquidLevel) -> Memory/1, LL1/1
  Control/1(LiquidIn) -> Logical Operator/1
  Control/2(LiquidOut) -> TankModel/2(LiquidOut)
  Memory/1 -> Control/4(LiquidLevel), MasterTankControl/1(LiquidTank1)
  MR1/1 -> Control/2(ManualReference)
  CT1/1 -> Control/1(ControlType)
  Memory1/1 -> MasterTankControl/2(LiquidTank2)
  EB1/1 -> Control/3(EmergencyButton)
  MasterTankControl/1(AllowTheTankFilling) -> Logical Operator/2
  Logical Operator/1 -> TankModel/1(LiquidIn)
  LL2/1 -> Memory1/1

== system c00009M_harness/M111/Tank2 ==
  CT2 : Inport
  MR2 : Inport  Port=2
  T2 : Inport  Port=3
  EB2 : Inport  Port=4
  LL1 : Inport  Port=5
  Control : Subsystem
  Logical Operator : Logic  AllPortsSameDT=off  OutDataTypeStr=boolean
  MasterTankControl : Subsystem
  Memory : Memory
  Memory1 : Memory
  TankModel : Subsystem
  LL2 : Outport
  wires:
  TankModel/1(LiquidLevel) -> Memory/1, LL2/1
  Control/1(LiquidIn) -> Logical Operator/1
  Control/2(LiquidOut) -> TankModel/2(LiquidOut)
  Memory/1 -> Control/5(LiquidLevel), MasterTankControl/2(LiquidTank2)
  MR2/1 -> Control/3(ManualReference)
  CT2/1 -> Control/2(StartMaintenance), Control/1(ControlType)
  Memory1/1 -> MasterTankControl/1(LiquidTank1)
  EB2/1 -> Control/4(EmergencyButton)
  MasterTankControl/1(AllowTheTankFilling) -> Logical Operator/2
  Logical Operator/1 -> TankModel/1(LiquidIn)
  LL1/1 -> Memory1/1

== system c00009M_harness/M112/Tank1 ==
  CT1 : Inport
  MR1 : Inport  Port=2
  T1 : Inport  Port=3
  EB1 : Inport  Port=4
  LL2 : Inport  Port=5
  Control : Subsystem
  Logical Operator : Logic  AllPortsSameDT=off  OutDataTypeStr=boolean
  MasterTankControl : Subsystem
  Memory : Memory
  Memory1 : Memory
  TankModel : Subsystem
  LL1 : Outport
  wires:
  TankModel/1(LiquidLevel) -> Memory/1, LL1/1
  Control/1(LiquidIn) -> Logical Operator/1
  Control/2(LiquidOut) -> TankModel/2(LiquidOut)
  Memory/1 -> Control/4(LiquidLevel), MasterTankControl/1(LiquidTank1)
  MR1/1 -> Control/2(ManualReference)
  CT1/1 -> Control/1(ControlType)
  Memory1/1 -> MasterTankControl/2(LiquidTank2)
  EB1/1 -> Control/3(EmergencyButton)
  MasterTankControl/1(AllowTheTankFilling) -> Logical Operator/2
  Logical Operator/1 -> TankModel/1(LiquidIn)
  LL2/1 -> Memory1/1

== system c00009M_harness/M112/Tank2 ==
  CT2 : Inport
  MR2 : Inport  Port=2
  T2 : Inport  Port=3
  EB2 : Inport  Port=4
  LL1 : Inport  Port=5
  Control : Subsystem
  Logical Operator : Logic  AllPortsSameDT=off  OutDataTypeStr=boolean
  MasterTankControl : Subsystem
  Memory : Memory
  Memory1 : Memory
  TankModel : Subsystem
  LL2 : Outport
  wires:
  TankModel/1(LiquidLevel) -> Memory/1, LL2/1
  Control/1(LiquidIn) -> Logical Operator/1
  Control/2(LiquidOut) -> TankModel/2(LiquidOut)
  Memory/1 -> Control/5(LiquidLevel), MasterTankControl/2(LiquidTank2)
  MR2/1 -> Control/3(ManualReference)
  CT2/1 -> Control/2(StartMaintenance), Control/1(ControlType)
  Memory1/1 -> MasterTankControl/1(LiquidTank1)
  EB2/1 -> Control/4(EmergencyButton)
  MasterTankControl/1(AllowTheTankFilling) -> Logical Operator/2
  Logical Operator/1 -> TankModel/1(LiquidIn)
  LL1/1 -> Memory1/1

== system c00009M_harness/M113/Tank1 ==
  CT1 : Inport
  MR1 : Inport  Port=2
  T1 : Inport  Port=3
  EB1 : Inport  Port=4
  LL2 : Inport  Port=5
  Control : Subsystem
  Logical Operator : Logic  AllPortsSameDT=off  OutDataTypeStr=boolean
  MasterTankControl : Subsystem
  Memory : Memory
  Memory1 : Memory
  TankModel : Subsystem
  LL1 : Outport
  wires:
  TankModel/1(LiquidLevel) -> Memory/1, LL1/1
  Control/1(LiquidIn) -> Logical Operator/1
  Control/2(LiquidOut) -> TankModel/2(LiquidOut)
  Memory/1 -> Control/4(LiquidLevel), MasterTankControl/1(LiquidTank1)
  MR1/1 -> Control/2(ManualReference)
  CT1/1 -> Control/1(ControlType)
  Memory1/1 -> MasterTankControl/2(LiquidTank2)
  EB1/1 -> Control/3(EmergencyButton)
  MasterTankControl/1(AllowTheTankFilling) -> Logical Operator/2
  Logical Operator/1 -> TankModel/1(LiquidIn)
  LL2/1 -> Memory1/1

== system c00009M_harness/M113/Tank2 ==
  CT2 : Inport
  MR2 : Inport  Port=2
  T2 : Inport  Port=3
  EB2 : Inport  Port=4
  LL1 : Inport  Port=5
  Control : Subsystem
  Logical Operator : Logic  AllPortsSameDT=off  OutDataTypeStr=boolean
  MasterTankControl : Subsystem
  Memory : Memory
  Memory1 : Memory
  TankModel : Subsystem
  LL2 : Outport
  wires:
  TankModel/1(LiquidLevel) -> Memory/1, LL2/1
  Control/1(LiquidIn) -> Logical Operator/1
  Control/2(LiquidOut) -> TankModel/2(LiquidOut)
  Memory/1 -> Control/5(LiquidLevel), MasterTankControl/2(LiquidTank2)
  MR2/1 -> Control/3(ManualReference)
  CT2/1 -> Control/2(StartMaintenance), Control/1(ControlType)
  Memory1/1 -> MasterTankControl/1(LiquidTank1)
  EB2/1 -> Control/4(EmergencyButton)
  MasterTankControl/1(AllowTheTankFilling) -> Logical Operator/2
  Logical Operator/1 -> TankModel/1(LiquidIn)
  LL1/1 -> Memory1/1

== system c00009M_harness/M114/Tank1 ==
  CT1 : Inport
  MR1 : Inport  Port=2
  T1 : Inport  Port=3
  EB1 : Inport  Port=4
  LL2 : Inport  Port=5
  Control : Subsystem
  Logical Operator : Logic  AllPortsSameDT=off  OutDataTypeStr=boolean
  MasterTankControl : Subsystem
  Memory : Memory
  Memory1 : Memory
  TankModel : Subsystem
  LL1 : Outport
  wires:
  TankModel/1(LiquidLevel) -> Memory/1, LL1/1
  Control/1(LiquidIn) -> Logical Operator/1
  Control/2(LiquidOut) -> TankModel/2(LiquidOut)
  Memory/1 -> Control/4(LiquidLevel), MasterTankControl/1(LiquidTank1)
  MR1/1 -> Control/2(ManualReference)
  CT1/1 -> Control/1(ControlType)
  Memory1/1 -> MasterTankControl/2(LiquidTank2)
  EB1/1 -> Control/3(EmergencyButton)
  MasterTankControl/1(AllowTheTankFilling) -> Logical Operator/2
  Logical Operator/1 -> TankModel/1(LiquidIn)
  LL2/1 -> Memory1/1

== system c00009M_harness/M114/Tank2 ==
  CT2 : Inport
  MR2 : Inport  Port=2
  T2 : Inport  Port=3
  EB2 : Inport  Port=4
  LL1 : Inport  Port=5
  Control : Subsystem
  Logical Operator : Logic  AllPortsSameDT=off  OutDataTypeStr=boolean
  MasterTankControl : Subsystem
  Memory : Memory
  Memory1 : Memory
  TankModel : Subsystem
  LL2 : Outport
  wires:
  TankModel/1(LiquidLevel) -> Memory/1, LL2/1
  Control/1(LiquidIn) -> Logical Operator/1
  Control/2(LiquidOut) -> TankModel/2(LiquidOut)
  Memory/1 -> Control/5(LiquidLevel), MasterTankControl/2(LiquidTank2)
  MR2/1 -> Control/3(ManualReference)
  CT2/1 -> Control/2(StartMaintenance), Control/1(ControlType)
  Memory1/1 -> MasterTankControl/1(LiquidTank1)
  EB2/1 -> Control/4(EmergencyButton)
  MasterTankControl/1(AllowTheTankFilling) -> Logical Operator/2
  Logical Operator/1 -> TankModel/1(LiquidIn)
  LL1/1 -> Memory1/1

== system c00009M_harness/M115/Tank1 ==
  CT1 : Inport
  MR1 : Inport  Port=2
  T1 : Inport  Port=3
  EB1 : Inport  Port=4
  LL2 : Inport  Port=5
  Control : Subsystem
  Logical Operator : Logic  AllPortsSameDT=off  OutDataTypeStr=boolean
  MasterTankControl : Subsystem
  Memory : Memory
  Memory1 : Memory
  TankModel : Subsystem
  LL1 : Outport
  wires:
  TankModel/1(LiquidLevel) -> Memory/1, LL1/1
  Control/1(LiquidIn) -> Logical Operator/1
  Control/2(LiquidOut) -> TankModel/2(LiquidOut)
  Memory/1 -> Control/4(LiquidLevel), MasterTankControl/1(LiquidTank1)
  MR1/1 -> Control/2(ManualReference)
  CT1/1 -> Control/1(ControlType)
  Memory1/1 -> MasterTankControl/2(LiquidTank2)
  EB1/1 -> Control/3(EmergencyButton)
  MasterTankControl/1(AllowTheTankFilling) -> Logical Operator/2
  Logical Operator/1 -> TankModel/1(LiquidIn)
  LL2/1 -> Memory1/1

== system c00009M_harness/M115/Tank2 ==
  CT2 : Inport
  MR2 : Inport  Port=2
  T2 : Inport  Port=3
  EB2 : Inport  Port=4
  LL1 : Inport  Port=5
  Control : Subsystem
  Logical Operator : Logic  AllPortsSameDT=off  OutDataTypeStr=boolean
  MasterTankControl : Subsystem
  Memory : Memory
  Memory1 : Memory
  TankModel : Subsystem
  LL2 : Outport
  wires:
  TankModel/1(LiquidLevel) -> Memory/1, LL2/1
  Control/1(LiquidIn) -> Logical Operator/1
  Control/2(LiquidOut) -> TankModel/2(LiquidOut)
  Memory/1 -> Control/5(LiquidLevel), MasterTankControl/2(LiquidTank2)
  MR2/1 -> Control/3(ManualReference)
  CT2/1 -> Control/2(StartMaintenance), Control/1(ControlType)
  Memory1/1 -> MasterTankControl/1(LiquidTank1)
  EB2/1 -> Control/4(EmergencyButton)
  MasterTankControl/1(AllowTheTankFilling) -> Logical Operator/2
  Logical Operator/1 -> TankModel/1(LiquidIn)
  LL1/1 -> Memory1/1

== system c00009M_harness/M116/Tank1 ==
  CT1 : Inport
  MR1 : Inport  Port=2
  T1 : Inport  Port=3
  EB1 : Inport  Port=4
  LL2 : Inport  Port=5
  Control : Subsystem
  Logical Operator : Logic  AllPortsSameDT=off  OutDataTypeStr=boolean
  MasterTankControl : Subsystem
  Memory : Memory
  Memory1 : Memory
  TankModel : Subsystem
  LL1 : Outport
  wires:
  TankModel/1(LiquidLevel) -> Memory/1, LL1/1
  Control/1(LiquidIn) -> Logical Operator/1
  Control/2(LiquidOut) -> TankModel/2(LiquidOut)
  Memory/1 -> Control/4(LiquidLevel), MasterTankControl/1(LiquidTank1)
  MR1/1 -> Control/2(ManualReference)
  CT1/1 -> Control/1(ControlType)
  Memory1/1 -> MasterTankControl/2(LiquidTank2)
  EB1/1 -> Control/3(EmergencyButton)
  MasterTankControl/1(AllowTheTankFilling) -> Logical Operator/2
  Logical Operator/1 -> TankModel/1(LiquidIn)
  LL2/1 -> Memory1/1

== system c00009M_harness/M116/Tank2 ==
  CT2 : Inport
  MR2 : Inport  Port=2
  T2 : Inport  Port=3
  EB2 : Inport  Port=4
  LL1 : Inport  Port=5
  Control : Subsystem
  Logical Operator : Logic  AllPortsSameDT=off  OutDataTypeStr=boolean
  MasterTankControl : Subsystem
  Memory : Memory
  Memory1 : Memory
  TankModel : Subsystem
  LL2 : Outport
  wires:
  TankModel/1(LiquidLevel) -> Memory/1, LL2/1
  Control/1(LiquidIn) -> Logical Operator/1
  Control/2(LiquidOut) -> TankModel/2(LiquidOut)
  Memory/1 -> Control/5(LiquidLevel), MasterTankControl/2(LiquidTank2)
  MR2/1 -> Control/3(ManualReference)
  CT2/1 -> Control/2(StartMaintenance), Control/1(ControlType)
  Memory1/1 -> MasterTankControl/1(LiquidTank1)
  EB2/1 -> Control/4(EmergencyButton)
  MasterTankControl/1(AllowTheTankFilling) -> Logical Operator/2
  Logical Operator/1 -> TankModel/1(LiquidIn)
  LL1/1 -> Memory1/1

== system c00009M_harness/M117/Tank1 ==
  CT1 : Inport
  MR1 : Inport  Port=2
  T1 : Inport  Port=3
  EB1 : Inport  Port=4
  LL2 : Inport  Port=5
  Control : Subsystem
  Logical Operator : Logic  AllPortsSameDT=off  OutDataTypeStr=boolean
  MasterTankControl : Subsystem
  Memory : Memory
  Memory1 : Memory
  TankModel : Subsystem
  LL1 : Outport
  wires:
  TankModel/1(LiquidLevel) -> Memory/1, LL1/1
  Control/1(LiquidIn) -> Logical Operator/1
  Control/2(LiquidOut) -> TankModel/2(LiquidOut)
  Memory/1 -> Control/4(LiquidLevel), MasterTankControl/1(LiquidTank1)
  MR1/1 -> Control/2(ManualReference)
  CT1/1 -> Control/1(ControlType)
  Memory1/1 -> MasterTankControl/2(LiquidTank2)
  EB1/1 -> Control/3(EmergencyButton)
  MasterTankControl/1(AllowTheTankFilling) -> Logical Operator/2
  Logical Operator/1 -> TankModel/1(LiquidIn)
  LL2/1 -> Memory1/1

== system c00009M_harness/M117/Tank2 ==
  CT2 : Inport
  MR2 : Inport  Port=2
  T2 : Inport  Port=3
  EB2 : Inport  Port=4
  LL1 : Inport  Port=5
  Control : Subsystem
  Logical Operator : Logic  AllPortsSameDT=off  OutDataTypeStr=boolean
  MasterTankControl : Subsystem
  Memory : Memory
  Memory1 : Memory
  TankModel : Subsystem
  LL2 : Outport
  wires:
  TankModel/1(LiquidLevel) -> Memory/1, LL2/1
  Control/1(LiquidIn) -> Logical Operator/1
  Control/2(LiquidOut) -> TankModel/2(LiquidOut)
  Memory/1 -> Control/5(LiquidLevel), MasterTankControl/2(LiquidTank2)
  MR2/1 -> Control/3(ManualReference)
  CT2/1 -> Control/2(StartMaintenance), Control/1(ControlType)
  Memory1/1 -> MasterTankControl/1(LiquidTank1)
  EB2/1 -> Control/4(EmergencyButton)
  MasterTankControl/1(AllowTheTankFilling) -> Logical Operator/2
  Logical Operator/1 -> TankModel/1(LiquidIn)
  LL1/1 -> Memory1/1

== system c00009M_harness/M128/Tank1 ==
  CT1 : Inport
  MR1 : Inport  Port=2
  T1 : Inport  Port=3
  EB1 : Inport  Port=4
  LL2 : Inport  Port=5
  Control : Subsystem
  Logical Operator : Logic  AllPortsSameDT=off  OutDataTypeStr=boolean
  MasterTankControl : Subsystem
  Memory : Memory
  Memory1 : Memory
  TankModel : Subsystem
  LL1 : Outport
  wires:
  TankModel/1(LiquidLevel) -> Memory/1, LL1/1
  Control/1(LiquidIn) -> Logical Operator/1
  Control/2(LiquidOut) -> TankModel/2(LiquidOut)
  Memory/1 -> Control/4(LiquidLevel), MasterTankControl/1(LiquidTank1)
  MR1/1 -> Control/2(ManualReference)
  CT1/1 -> Control/1(ControlType)
  Memory1/1 -> MasterTankControl/2(LiquidTank2)
  EB1/1 -> Control/3(EmergencyButton)
  MasterTankControl/1(AllowTheTankFilling) -> Logical Operator/2
  Logical Operator/1 -> TankModel/1(LiquidIn)
  LL2/1 -> Memory1/1

== system c00009M_harness/M128/Tank2 ==
  CT2 : Inport
  MR2 : Inport  Port=2
  T2 : Inport  Port=3
  EB2 : Inport  Port=4
  LL1 : Inport  Port=5
  Control : Subsystem
  Logical Operator : Logic  AllPortsSameDT=off  OutDataTypeStr=boolean
  MasterTankControl : Subsystem
  Memory : Memory
  Memory1 : Memory
  TankModel : Subsystem
  LL2 : Outport
  wires:
  TankModel/1(LiquidLevel) -> Memory/1, LL2/1
  Control/1(LiquidIn) -> Logical Operator/1
  Control/2(LiquidOut) -> TankModel/2(LiquidOut)
  Memory/1 -> Control/5(LiquidLevel), MasterTankControl/2(LiquidTank2)
  MR2/1 -> Control/3(ManualReference)
  CT2/1 -> Control/2(StartMaintenance), Control/1(ControlType)
  Memory1/1 -> MasterTankControl/1(LiquidTank1)
  EB2/1 -> Control/4(EmergencyButton)
  MasterTankControl/1(AllowTheTankFilling) -> Logical Operator/2
  Logical Operator/1 -> TankModel/1(LiquidIn)
  LL1/1 -> Memory1/1
